simulink model "BalancedCar1"  (R2019b)
settings: Solver=VariableStepAuto  StartTime=0.0  StopTime=200  RelTol=1e-3
values from neighbouring files (symbols this model uses):
  A = sys_d.a    [LQRControler_DampingSystem.m]    (also in LQRControler_DampingSystem_TrajControl1.m; LQRControler_DampingSystem_TrajControl2.m; LQRControler_DampingSystem_TrajControl3.m; LQRController_BalanceCar.m)
  B = sys_d.b    [LQRControler_DampingSystem.m]    (also in LQRControler_DampingSystem_TrajControl1.m; LQRControler_DampingSystem_TrajControl2.m; LQRControler_DampingSystem_TrajControl3.m; LQRController_BalanceCar.m)
  F = F_N_min_k    (= inf)    [F1_LQR_Gain.m]    (also in LQRControler_DampingSystem.m = F1_LQR_Gain(A, B, Q, R, S); LQRControler_DampingSystem_TrajControl1.m = F1_LQR_Gain(Aa, Ba, Qa, R, Sa); LQRControler_DampingSystem_TrajControl2.m = F1_LQR_Gain(Aa, Ba, Qa, R, Sa); LQRControler_DampingSystem_TrajControl3.m = F1_LQR_Gain(Aa, Ba, Qa, R, Sa))
  x = A*x + B*u    [LQRControler_DampingSystem.m]    (also in LQRControler_DampingSystem_TrajControl1.m; LQRControler_DampingSystem_TrajControl2.m; LQRControler_DampingSystem_TrajControl3.m; LQRController_BalanceCar.m)
  x0 = [1 ; 0]    [LQRControler_DampingSystem.m]    (also in LQRControler_DampingSystem_TrajControl1.m = [0 ; 0]; LQRControler_DampingSystem_TrajControl2.m = [0 ; 0]; LQRControler_DampingSystem_TrajControl3.m = [0 ; 0]; LQRController_BalanceCar.m = [pi/180;0])
  xd = [1; 0]    [LQRControler_DampingSystem_TrajControl1.m]    (also in LQRControler_DampingSystem_TrajControl2.m; LQRControler_DampingSystem_TrajControl3.m = AD*xd; LQRController_BalanceCar.m = [0;0]; LQRController_BalanceCar1.m = [0; 0; 0; 0])
settings Model: Creator=ZHAO TAO  LastModifiedBy=ZHAO TAO

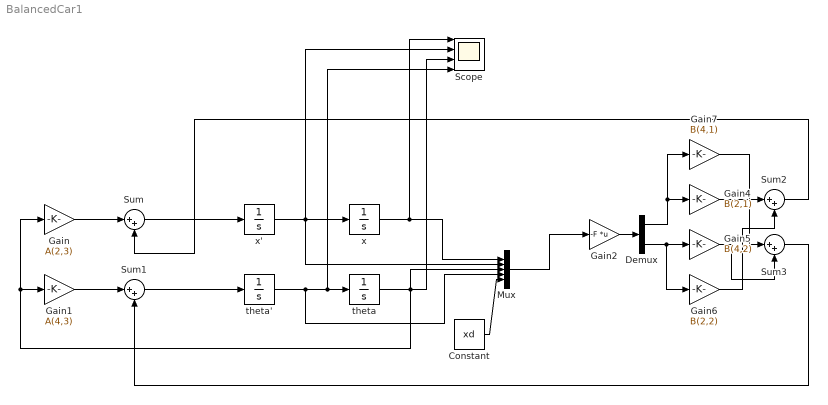
== system BalancedCar1 ==
  Constant : Constant  Value=xd
  Demux : Demux  Outputs=2
  Gain : Gain  Gain=A(2,3)
  Gain1 : Gain  Gain=A(4,3)
  Gain2 : Gain  Gain=-F  Multiplication=Matrix(K*u)
  Gain4 : Gain  Gain=B(2,1)
  Gain5 : Gain  Gain=B(4,2)
  Gain6 : Gain  Gain=B(2,2)
  Gain7 : Gain  Gain=B(4,1)
  Mux : Mux  Inputs=5
  Scope : Scope  NumInputPorts=4
  Sum{,1..3} (4 alike) : Sum  Inputs=|++
  theta : Integrator  InitialCondition=x0(3,1)
  theta' : Integrator  InitialCondition=x0(4,1)
  x : Integrator  InitialCondition=x(1,1)
  x' : Integrator  InitialCondition=x(2,1)
  wires:
  x'/1 -> Scope/2, Mux/2, x/1
  theta'/1 -> Scope/4, theta/1, Mux/4
  Sum/1 -> x'/1
  Sum1/1 -> theta'/1
  theta/1 -> Scope/3, Mux/3, Gain/1, Gain1/1
  Gain/1 -> Sum/1
  Gain1/1 -> Sum1/1
  x/1 -> Scope/1, Mux/1
  Gain4/1 -> Sum2/1
  Gain6/1 -> Sum2/2
  Gain5/1 -> Sum3/2
  Sum2/1 -> Sum/2
  Sum3/1 -> Sum1/2
  Mux/1 -> Gain2/1
  Gain2/1 -> Demux/1
  Demux/1 -> Gain7/1, Gain4/1
  Demux/2 -> Gain6/1, Gain5/1
  Gain7/1 -> Sum3/1
  Constant/1 -> Mux/5
